simulink model "fixedPoint_model_q3_c"  (R2020b)
settings: Solver=FixedStepDiscrete  StartTime=0.0  StopTime=10  FixedStep=1/44100  RelTol=1e-3  EnableMultiTasking=on
settings Model: SILPILModeSetting=veronly  ExtModeTrigDuration=2  Creator=Faridodin  LastModifiedBy=Faridodin
settings OptimizationCC: DefaultParameterBehavior=Inlined  EnhancedBackFolding=on  PassReuseOutputArgsAs=Individual arguments  ZeroExternalMemoryAtStartup=off  ZeroInternalMemoryAtStartup=off  OptimizeBlockOrder=speed  DifferentSizesBufferReuse=on  OptimizationCustomize=off  EfficientTunableParamExpr=on
settings DebuggingCC: ParameterTunabilityLossMsg=error
settings SFSimCC: MATLABDynamicMemAlloc=off
settings RTWCC: Description=Embedded Coder  SystemTargetFile=ert.tlc  TemplateMakefile=ert_default_tmf  BuildConfiguration=Faster Runs
settings CodeAppCC: ForceParamTrailComments=on  IgnoreCustomStorageClasses=off  OperatorAnnotations=on  SimulinkDataObjDesc=on  SFDataObjDesc=on  InsertBlockDesc=on
settings ERTTargetCC: TargetLangStandard=C99 (ISO)  GenerateSampleERTMain=on  InlinedParameterPlacement=NonHierarchical  ERTCustomFileTemplate=example_file_process.tlc

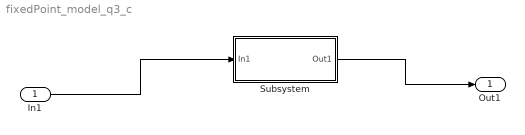
== system fixedPoint_model_q3_c ==
  In1 : Inport
  Subsystem : Subsystem
  Out1 : Outport
  wires:
  In1/1 -> Subsystem/1(In1)
  Subsystem/1(Out1) -> Out1/1

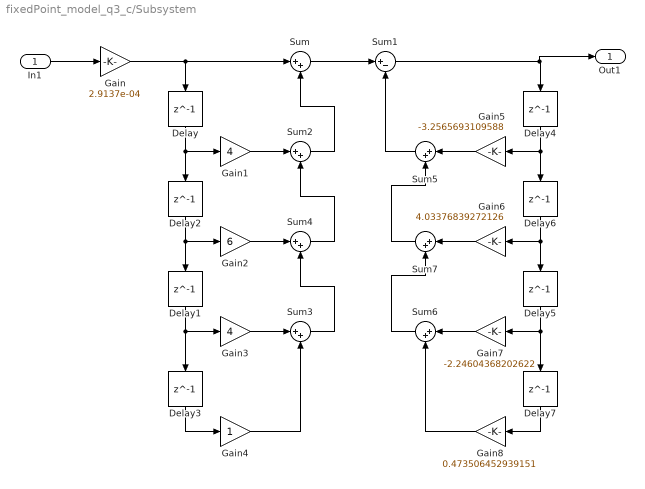
== system fixedPoint_model_q3_c/Subsystem ==
  In1 : Inport
  Delay{,1..7} (8 alike) : Delay  DelayLength=1  InitialCondition=0
  Gain : Gain  Gain=2.9137e-04
  Gain1 : Gain  Gain=4
  Gain2 : Gain  Gain=6
  Gain3 : Gain  Gain=4
  Gain4 : Gain
  Gain5 : Gain  Gain=-3.2565693109588
  Gain6 : Gain  Gain=4.03376839272126
  Gain7 : Gain  Gain=-2.24604368202622
  Gain8 : Gain  Gain=0.473506452939151
  Sum{,2..7} (7 alike) : Sum  Inputs=|++
  Sum1 : Sum  Inputs=|+-
  Out1 : Outport
  wires:
  Delay4/1 -> Delay6/1, Gain5/1
  Gain4/1 -> Sum3/2
  Sum5/1 -> Sum1/2
  Sum3/1 -> Sum4/2
  Delay7/1 -> Gain8/1
  Delay/1 -> Delay2/1, Gain1/1
  Delay3/1 -> Gain4/1
  Delay1/1 -> Delay3/1, Gain3/1
  Gain3/1 -> Sum3/1
  Sum1/1 -> Out1/1, Delay4/1
  Gain8/1 -> Sum6/2
  Gain7/1 -> Sum6/1
  Gain6/1 -> Sum7/1
  Sum6/1 -> Sum7/2
  Delay6/1 -> Delay5/1, Gain6/1
  Sum/1 -> Sum1/1
  Gain5/1 -> Sum5/1
  Delay2/1 -> Delay1/1, Gain2/1
  Sum4/1 -> Sum2/2
  Sum7/1 -> Sum5/2
  Gain2/1 -> Sum4/1
  Gain/1 -> Sum/1, Delay/1
  Sum2/1 -> Sum/2
  Gain1/1 -> Sum2/1
  Delay5/1 -> Delay7/1, Gain7/1
  In1/1 -> Gain/1
